simulink model "MotorSim"  (R2023b)
settings: Solver=VariableStepDiscrete  StartTime=0.0  StopTime=10.0  RelTol=1e-3
settings Model: Creator=YXuan  LastModifiedBy=YXuan
settings SolverCC: ZeroCrossControl=DisableAll  PositivePriorityOrder=on  AutoInsertRateTranBlk=on
settings OptimizationCC: DefaultUnderspecifiedDataType=single

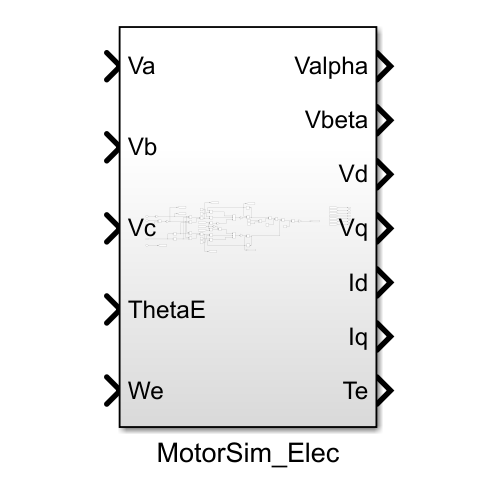
[thumbnail: Simulink's stored preview of the top-level diagram]
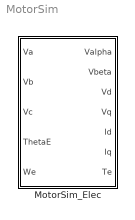
== system MotorSim ==
  MotorSim_Elec : Subsystem

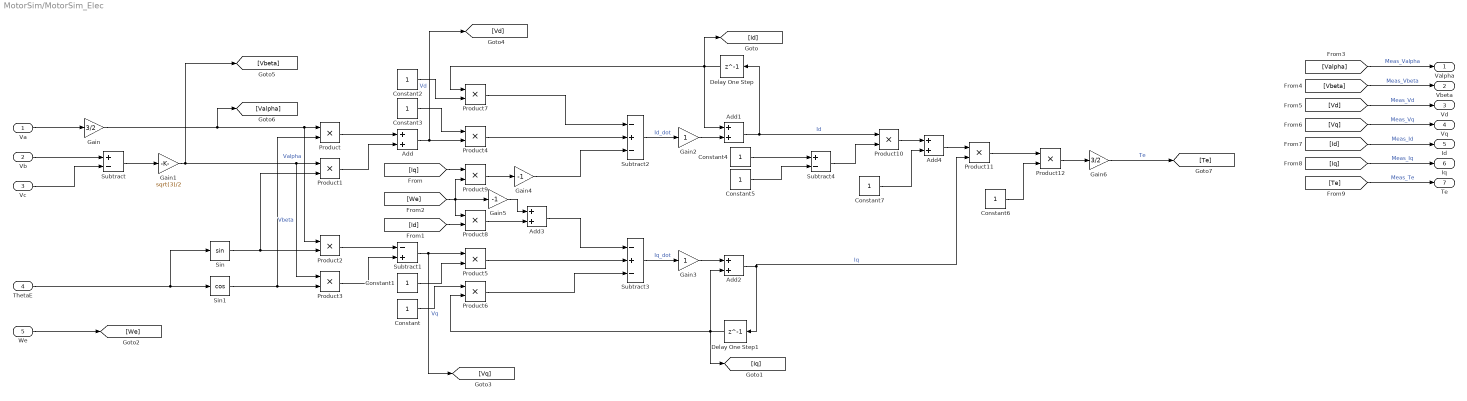
== system MotorSim/MotorSim_Elec ==
  Va : Inport
  Vb : Inport  Port=2
  Vc : Inport  Port=3
  ThetaE : Inport  Port=4
  We : Inport  Port=5
  Add{,1..4} (5 alike) : Sum
  Constant{,1..7} (8 alike) : Constant
  Delay One Step : Delay  DelayLength=1
  Delay One Step1 : Delay  DelayLength=1
  Gain : Gain  Gain=3/2
  Gain1 : Gain  Gain=sqrt(3)/2
  Gain2 : Gain
  Gain3 : Gain
  Gain4 : Gain  Gain=-1
  Gain5 : Gain  Gain=-1
  Gain6 : Gain  Gain=3/2
  Product{,1..12} (13 alike) : Product
  Sin : Trigonometry
  Sin1 : Trigonometry  Operator=cos
  Subtract : Sum  Inputs=+-
  Subtract1 : Sum  Inputs=-+
  Subtract2 : Sum  Inputs=-+-
  Subtract3 : Sum  Inputs=-+-
  Subtract4 : Sum  Inputs=+-
  Valpha : Outport
  Vbeta : Outport  Port=2
  Vd : Outport  Port=3
  Vq : Outport  Port=4
  Id : Outport  Port=5
  Iq : Outport  Port=6
  Te : Outport  Port=7
  wires:
  Product5/1 -> Subtract3/2
  Product2/1 -> Subtract1/1
  Gain3/1 -> Add2/1
  ThetaE/1 -> Sin/1, Sin1/1
  Subtract1/1 -> [Vq], Product5/1  "Vq"
  Gain/1 -> [Valpha], Product2/1, Product/1  "Valpha"
  Add4/1 -> Product11/1
  Constant5/1 -> Subtract4/2
  Delay One Step1/1 -> [Iq], Product6/2, Add2/2
  [Te] -> Te/1  "Meas_Te"
  Delay One Step/1 -> [Id], Product7/1, Add1/1
  Gain6/1 -> [Te]  "Te"
  [Vq] -> Vq/1  "Meas_Vq"
  Subtract/1 -> Gain1/1
  Sin/1 -> Product1/2, Product2/2
  [We] -> Gain5/1, Product9/2, Product8/1
  Gain4/1 -> Subtract2/3
  Product6/1 -> Subtract3/3
  Constant2/1 -> Product7/2
  Gain2/1 -> Add1/2
  [Id] -> Product8/2
  Add2/1 -> Product11/2, Delay One Step1/1  "Iq"
  Constant6/1 -> Product12/2
  Constant/1 -> Product6/1
  Add/1 -> [Vd], Product4/2  "Vd"
  Sin1/1 -> Product/2, Product3/2
  Product10/1 -> Add4/1
  Add1/1 -> Product10/1, Delay One Step/1  "Id"
  Product3/1 -> Subtract1/2
  [Iq] -> Iq/1  "Meas_Iq"
  Product/1 -> Add/1
  Constant3/1 -> Product4/1
  Constant1/1 -> Product5/2
  We/1 -> [We]
  Vb/1 -> Subtract/1
  Add3/1 -> Subtract3/1
  Product11/1 -> Product12/1
  Subtract3/1 -> Gain3/1  "Iq_dot"
  Product4/1 -> Subtract2/2
  Product1/1 -> Add/2
  Product12/1 -> Gain6/1
  Gain1/1 -> [Vbeta], Product3/1, Product1/1  "Vbeta"
  Product9/1 -> Gain4/1
  Gain5/1 -> Add3/1
  Product7/1 -> Subtract2/1
  Va/1 -> Gain/1
  [Valpha] -> Valpha/1  "Meas_Valpha"
  Constant4/1 -> Subtract4/1
  [Iq] -> Product9/1
  Vc/1 -> Subtract/2
  Subtract2/1 -> Gain2/1  "Id_dot"
  Constant7/1 -> Add4/2
  Product8/1 -> Add3/2
  Subtract4/1 -> Product10/2
  [Vbeta] -> Vbeta/1  "Meas_Vbeta"
  [Id] -> Id/1  "Meas_Id"
  [Vd] -> Vd/1  "Meas_Vd"
